simulink model "E102DigitalControllerP4"  (R2025a)
settings: Solver=VariableStepAuto  StartTime=0.0  StopTime=10.0  RelTol=1e-3
undefined symbols (not defined in the file or in its folder): dspblkCoreblockFVToolHelper, gcbh
settings Model: Creator=silva  LastModifiedBy=silva

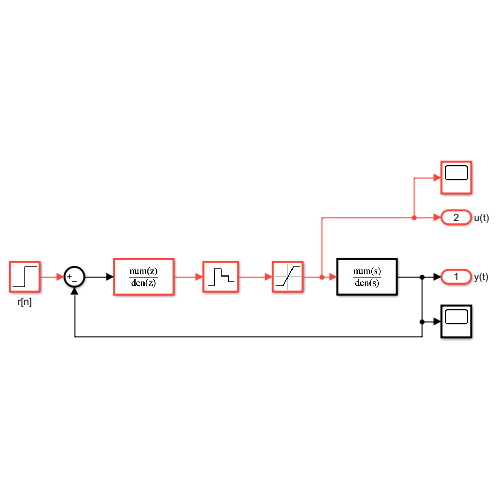
[thumbnail: Simulink's stored preview of the top-level diagram]
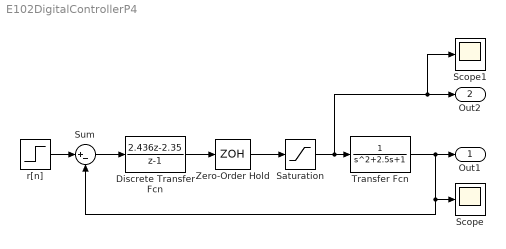
== system E102DigitalControllerP4 ==
  Discrete Transfer Fcn : DiscreteTransferFcn  LoadFcn=dspblkCoreblockFVToolHelper(gcbh,'load');  Numerator=[2.436 -2.35]  Denominator=[1 -1]
      settings: CopyFcn=dspblkCoreblockFVToolHelper(gcbh,'copy');  DeleteFcn=dspblkCoreblockFVToolHelper(gcbh,'close');  ModelCloseFcn=dspblkCoreblockFVToolHelper(gcbh,'close');  PreSaveFcn=dspblkCoreblockFVToolHelper(gcbh,'presave');  PostSaveFcn=dspblkCoreblockFVToolHelper(gcbh,'postsave');  CloseFcn=dspblkCoreblockFVToolHelper(gcbh,'close');
  Saturation : Saturate  UpperLimit=5  LowerLimit=0
  Scope : Scope
      settings: ActiveDisplayYMinimum=-1  ActiveDisplayYMaximum=1
  Scope1 : Scope
      settings: ActiveDisplayYMinimum=1.8552610100483307  ActiveDisplayYMaximum=5.3494154433279633
  Sum : Sum  Inputs=|+-
  Transfer Fcn : TransferFcn  Denominator=[1 2.5 1]
  Zero-Order Hold : ZeroOrderHold  SampleTime=0.1
  r[n] : Step  Time=0  After=2.5  SampleTime=0.1
  Out1 : Outport  SignalName=y(t)  SampleTime=0.1
  Out2 : Outport  Port=2  SignalName=u(t)  SampleTime=0.1
  wires:
  r[n]/1 -> Sum/1
  Zero-Order Hold/1 -> Saturation/1
  Sum/1 -> Discrete Transfer Fcn/1
  Discrete Transfer Fcn/1 -> Zero-Order Hold/1
  Saturation/1 -> Scope1/1, Out2/1, Transfer Fcn/1
  Transfer Fcn/1 -> Scope/1, Sum/2, Out1/1
